simulink model "F16ASYM_Controlled"  (R2015a)
settings: Solver=ode3  SolverMode=SingleTasking  StartTime=0.0  StopTime=inf  FixedStep=T_sim  RelTol=1e-3
InitFcn:
  | load('NN_c_weights_Last_stable.mat')
StopFcn:
  | Final_results
values from neighbouring files (symbols this model uses):
  a1 = fitresult.p1    [Stall_protection.m]
  alpha_map_eval = ones(size(M_eval))*NaN    [Auto_trim_aid.m]    (also in Autotrim_maps.mat = [nan nan 0.277598136245 0.119432432992 0.0579479097061 0.027)
  beta_map_eval = ones(size(M_eval))*NaN    [Auto_trim_aid.m]    (also in Autotrim_maps.mat = [nan nan -0.00151549403324 0.00117807579006 -0.0052086799721)
  C_L_0 = fitresult.p2    [Stall_protection.m]
  G_eval = NaN*ones(size(M_sq,2),size(H_sq,2))    [Stall_protection.m]
  H_sq = unique(sort(H_sq))    [Stall_protection.m]
  H_sq_autotrim = min( F_envelope.H_1g):2000:max(F_envelope.H_1g)    [Auto_trim_aid.m]    (also in Autotrim_maps.mat = [0 2000 4000 6000 8000 10000 12000 14000 16000 18000])
  K_b_q_extrap_ACC = K_b_q_extrap    [RUN_ME.m]
  K_b_q_extrap_AoA = K_b_q_extrap    [RUN_ME.m]
  M_sq = unique(sort(M_sq))    [Stall_protection.m]
  M_sq_autotrim = 0:0.1:max(F_envelope.M_1g)    [Auto_trim_aid.m]    (also in Autotrim_maps.mat = [0 0.1 0.2 0.3 0.4 0.5 0.6 0.7 0.8 0.9 1 1.1 ... (21 element)
  T_sim = 0.02    [RUN_ME.m]
  tau_q_extrap_ACC = tau_q_extrap    [RUN_ME.m]
  tau_q_extrap_AoA = tau_q_extrap    [RUN_ME.m]
  velocity = M_eval(I,J)*a    [Auto_trim_aid.m]
undefined symbols (not defined in the file or in its folder): ACCEL, B, Earth, fi_flag_Simulink, GYRO, H_sq_sche, k_B, K_b_ACC_extrap, K_b_AoA_extrap, latitude, longitude, m, m_B, M_sq_sche, Model_used_flag, rad, s, sigbuilder_block, Stall_curve, tau_ACC_extrap, tau_AoA_extrap, Theta_1_roll_last, Theta_2_roll_last, Theta_3_roll_last, trim_control, trim_state, trim_throttle, V_Comp_A_w_z_last, V_Comp_last, V_Comp_last_ONE, V_long_lastA_w_z, V_long_lastAoA, V_roll_last, V_roll_lastMOD, V_yaw_last, W_Comp_A_w_z_last, W_Comp_last, W_long_lastA_w_z, W_long_lastAoA, W_roll_last, W_roll_lastMOD, W_yaw_last, WGS84
libraries: Adaptive_FaultTolerantControl x57, dspsigops x37, F16_Actuator_Library x14, commnoisgen2 x13, simulink x11, simulink_extras x10, dsparch4 x6, aerolibatmos2 x6, aerolibtransform2 x6, aerolibfltsims x3, dspvision x3, dspsnks4 x3
(part 1 of 14)
Description:
  | This models and controllers were implemented by David Torres Ocaña at Cranfield University
settings Model: ModifiedHistory=This models and controllers were implemented by David Torres Ocaña at Cranfield University  MAModelExclusionFile=C:\Users\David\Documents\Estudios y formación academica\Cranfield\Thesis F16\Work\Solutions\7dof Base\F16ASYM_Controlled_exclusions.xml  Creator=David  LastModifiedBy=david
settings SolverCC: AutoInsertRateTranBlk=on
settings DataIOCC: SaveOutput=off  SignalLogging=off  DSMLogging=off  SaveTime=off
settings OptimizationCC: BlockReduction=off  InlineParams=on  InlineInvariantSignals=on  EnableMemcpy=off  ExpressionDepthLimit=2147483647  StateBitsets=on  DataBitsets=on  ZeroExternalMemoryAtStartup=off  ZeroInternalMemoryAtStartup=off  NoFixptDivByZeroProtection=on  EfficientMapNaN2IntZero=off  OptimizeModelRefInitCode=on  LifeSpan=1
settings DebuggingCC: UnderspecifiedInitializationDetection=Classic  MergeDetectMultiDrivingBlocksExec=none  SolverPrmCheckMsg=warning  ParameterPrecisionLossMsg=none  StateNameClashWarn=warning
settings HardwareCC: ProdIntDivRoundTo=Floor  ProdEndianess=LittleEndian  ProdHWDeviceType=Generic->Custom
settings RTWCC: SystemTargetFile=ert.tlc  TLCOptions=-p0  GenCodeOnly=on  TemplateMakefile=ert_default_tmf  Description=Embedded Coder  GenerateReport=on  RTWVerbose=off  IncludeHyperlinkInReport=on  LaunchReport=on
settings CodeAppCC: ForceParamTrailComments=on  IgnoreCustomStorageClasses=off  SimulinkDataObjDesc=on  CustomSymbolStrGlobalVar=rt$N$M  CustomSymbolStrType=$N$M  CustomSymbolStrFcn=$N$M$F  CustomSymbolStrMacro=$N$M  InsertBlockDesc=on  InternalIdentifier=Classic
settings ERTTargetCC: TargetLangStandard=C99 (ISO)  ParMdlRefBuildCompliant=on  CompOptLevelCompliant=on  ConcurrentExecutionCompliant=on  IncludeMdlTerminateFcn=off  SuppressErrorStatus=on  ERTFirstTimeCompliant=on  SupportAbsoluteTime=off  SupportNonFinite=off  SupportComplex=off  PurelyIntegerCode=on  SupportContinuousTime=off  SupportVariableSizeSignals=off  ModelStepFunctionPrototypeControlCompliant=on  CPPClassGenCompliant=on  RootIOFormat=Structure reference  ERTCustomFileTemplate=example_file_process.tlc

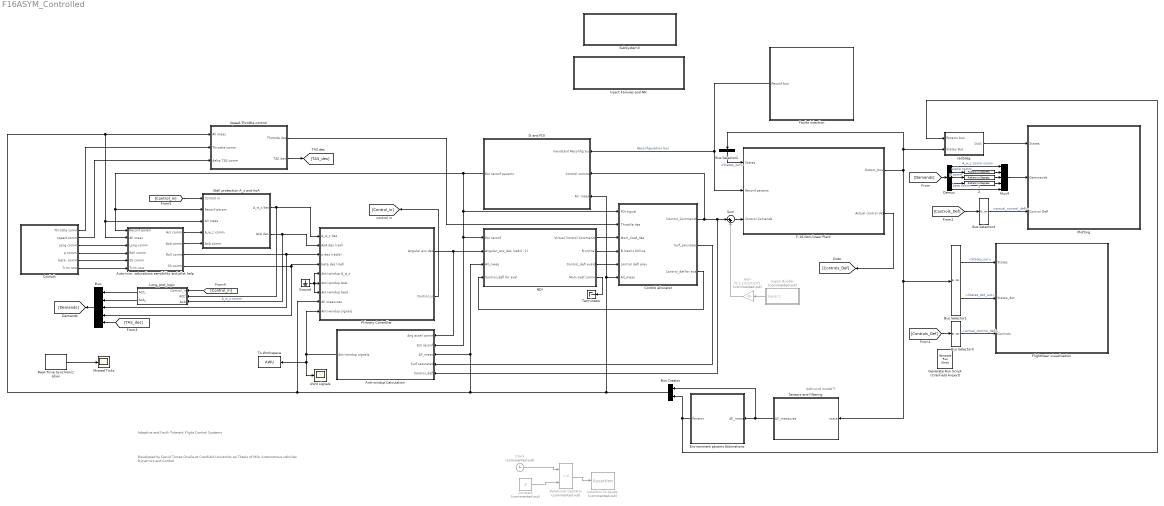
== system F16ASYM_Controlled ==
  note: Developed by David Torres Ocaña
      | at Cranfield University as Thesis of
      | MSc Autonomous vehicles Dynamics and Control
  note: Add wind model??
  note: Adaptive and Fault-Tolerant Flight Control Systems
  "  " : simulink_extras/Transformations/Radians to Degrees
  "  1" : simulink_extras/Transformations/Radians to Degrees
  "  2" : simulink_extras/Transformations/Radians to Degrees
  AWU signals : Scope
      settings: YMin=-30  YMax=15  SaveName=ScopeData20
  Anti-windup Calculation : Subsystem  Variant=on  OverrideUsingVariant=No reconfigurable
  Assertion to pause : Assertion  Commented=on  AssertionFailFcn=|  StopWhenAssertionFail=off
      | set_param(bdroot,'SimulationCommand','pause'),
      | disp(sprintf('\nSimulation paused.'))
  "Auto-trim, saturations sensibility and pilot help" : Subsystem
  Bus Creator : BusCreator  Inputs=2
  Bus Selector1 : BusSelector  OutputSignals=States_out,States_dot_out
  Bus Selector2 : BusSelector  OutputSignals=States_out
  Bus Selector3 : BusSelector  OutputSignals=actual_control_defl
  Bus Selector4 : BusSelector  OutputSignals=actual_control_defl
  Clock : Clock  Commented=on
  Cockpit : Subsystem
      mask Display:
      | image(imread('Cockpit2.jpg'))
      | 
      | port_label('output', 1, 'Throttle comm')
      | port_label('output', 2, 'Speed comm')
      | port_label('output', 3, 'Long comm')
      | port_label('output', 4, 'p comm')
      | port_label('output', 5, 'beta comm')
      | port_label('output', 6, 'Trim now')
  Constant : Constant  Commented=on  Value=5
  Control allocator : Subsystem  Variant=on  OverrideUsingVariant=Control Allocator: NO RECONFIG
  Demux : Demux  Outputs=5
  Environment params Estimations : Subsystem
  F-16 Non-linear Plant : Subsystem  Variant=on  OverrideUsingVariant=Reconfigurable
      mask Display:
      | image(imread('f16.jpg'))
      | 
      | port_label('output', 1, 'Out_bus')
      | port_label('output', 2, 'Actual Control deflec')
      | 
      | port_label('input', 1, 'State_feedback')
      | port_label('input', 2, 'Reconf_params')
      | port_label('input', 3, 'Control_Commands')
      | 
      | % Variant dealing
      | ActiveVar = get_param(gcb,'activevariant');
      | 
      | 
      | disp(['{\bf\fontsize{16}',ActiveVar,'}'], 'texmode','on');
  Faults injection : Subsystem
      settings: OpenFcn=Control_GUI
      mask Display: disp(['{\bf \fontsize{16}',sprintf('Faults \n and\n  deviations\n  injection'),'}'], 'texmode','on');
  FlightGear visualization : Subsystem  TreatAsAtomicUnit=on
      mask Display:
      | % disp('{\bf\fontsize{20} Flight Gear}', 'texmode','on');
      | image(imread('FG F16.jpg'))
      | % image(imread('FlightGear_logo.png'))
  Gain : Gain  Commented=on  Gain=[0,1,1,0,0,0,0,0]
  Generate Run Script (Cranfield Airport) : aerolibfltsims/Generate Run Script  OutputFileName=runfg.bat  FlightGearBaseDirectory=C:\Program Files\FlightGear  GeometryModelName=f16  DestinationPort=5502  OriginAddress=127.0.0.1  OriginPort=5505  LocalAddress=127.0.0.1  AirportId=EGTC  RunwayId=1  InitialAltitude=trim_state(3)*3.2808399  InitialHeading=0  OffsetDistance=4.72  OffsetAzimuth=0  GenerateFile=off  Architecture=Win64  dataFlow=Send
  Ground : Ground
  Inject Failures and NN : Subsystem
      settings: OpenFcn=Control_GUI
      mask Display: disp('Inject Failures & NN management GUI')
  Long_plot_logic : MATLAB Function  TreatAsAtomicUnit=on
  Missed Ticks : Scope
      settings: TickLabels=on  TimeRange=20  YMin=0  YMax=70  SaveName=ScopeData29
  Mux : Mux  Inputs=[1 1 1 1 1]
  Mux4 : Mux  Inputs=5
  NDI : Subsystem  Variant=on  OverrideUsingVariant=NDI: NO RECONFIG
  Plotting : Subsystem
      mask Display:
      | disp('{\bf\fontsize{20} Plotting}', 'texmode','on');
      | % port_label('input', 1, 'States')
      | % port_label('input', 2, 'Demans')
  Primary Controller : Subsystem  Variant=on  OverrideUsingVariant=Adaptive Controller Crossed+AWU+Lim
  Real-Time Synchronization : sldrtlib/Real-Time Synchronization  SampleTime=T_sim  MaxMissedTicks=100000  ShowMissedTicks=on  YieldWhenWaiting=on
  Relational Operator : RelationalOperator  Commented=on  Operator=~=  OutDataTypeStr=boolean
  SI and FDI : Subsystem  Variant=on  OverrideUsingVariant=Realistic
      mask Display:
      | % Variant dealing
      | ActiveVar = get_param(gcb,'activevariant');
      | 
      | 
      | 
      | disp(['{\bf \fontsize{14}',sprintf('SI \n&\nFDI\n\n '),ActiveVar,'}'], 'texmode','on');
  Sensors and filtering : Subsystem  Variant=on  OverrideUsingVariant=No noise
  Signal Builder : Subsystem  Tag=STV Subsys  Commented=on  LoadFcn=sigbuilder_block('load');  StartFcn=sigbuilder_block('start');  StopFcn=sigbuilder_block('stop');  ClipboardFcn=sigbuilder_block('clipboard');  mask(Sigbuilder block){}
      mask help: Simulink:masks:SigbuilderBlock_MD
      mask init:
      | if ~strcmp(get_param(bdroot(gcbh),'SimulationStatus'),'stopped') tuvar = sigbuilder_block('maskInit'); end
      settings: CopyFcn=sigbuilder_block('copy');  DeleteFcn=sigbuilder_block('delete');  ModelCloseFcn=sigbuilder_block('modelClose');  PreSaveFcn=sigbuilder_block('preSave');  PauseFcn=sigbuilder_block('pause');  ContinueFcn=sigbuilder_block('continue');  NameChangeFcn=sigbuilder_block('namechange');  OpenFcn=sigbuilder_block('open',[437.25 118.5 550.5 394.5 ]);  CloseFcn=sigbuilder_block('close');
      mask Display: plot(0, 0, 100, 100,[2, 2, 32, 32, 2], [68, 8, 8, 68, 68],[32, 2], [38, 38], [32, 19, 2],[53, 60, 44], [32, 17, 17, 2],[16, 16, 31, 31]);txt = getActiveGroup(gcbh);text(2, 100, txt,'verticalAlignment', 'top');
  Speed-Throttle control : Subsystem
  Stall protection A_z and AoA : Subsystem  Variant=on  OverrideUsingVariant=Using AoA
  SubSystem3 : Subsystem
      settings: OpenFcn=FE_plot
      mask Display:
      | % image(imread('FE.png'))
      | 
      | disp('Flight Envelope position');
  Sum : Sum  Inputs=|++
  Terminator : Terminator
  To Workspace : ToWorkspace  VariableName=AWU  SaveFormat=Timeseries  SampleTime=-1
  rad2deg : Subsystem
  wires:
  rad2deg/1(Out1) -> Plotting/1(States)
  F-16 Non-linear Plant/1(Output_bus) -> Bus Selector1/1, Sensors and filtering/1(state), Bus Selector2/1, rad2deg/2(States Bus)
  Bus Selector1/1 -> FlightGear visualization/1(States)  "<States_out>"
  Bus Selector1/2 -> FlightGear visualization/2(States_dot)  "<States_dot_out>"
  [Demands] -> Demux/1
  Sensors and filtering/1(All_measures) -> Bus Creator/1, Environment params Estimations/1(All_meas)
  Environment params Estimations/1(Params) -> Bus Creator/2, rad2deg/1(Params bus)
  Demux/3 -> "  1"/1  "p comm"
  Demux/4 -> "  2"/1  "beta comm"
  Demux/2 -> "  "/1  "alpha comm"
  [Controls_Def] -> Bus Selector3/1
  Control allocator/2(Surf_saturated) -> Anti-windup Calculation/4(Surf saturated)
  NDI/1(Virtual Control Commands) -> Control allocator/3(Mom_Coef_des)
  Ground/1 -> Primary Controller/7(Anti-windup beta), Primary Controller/5(Anti-windup A_w_z), Primary Controller/6(Anti-windup AoA)
  Mux4/1 -> Plotting/2(Demmands)
  Bus Selector2/1 -> F-16 Non-linear Plant/1(States)  "<States_out>"
  NDI/2(B online) -> Control allocator/4(B matrix Online)
  Demux/1 -> Mux4/1  "A_w_z comm comm"
  "  "/1 -> Mux4/2
  "  1"/1 -> Mux4/3
  "  2"/1 -> Mux4/4
  F-16 Non-linear Plant/2(Actual control def) -> [Controls_Def]
  Bus Selector3/1 -> FlightGear visualization/3(Controls)  "<actual_control_defl>"
  Primary Controller/1(Angular acc des) -> NDI/2(Angular_acc_des (rad/s^2)), Anti-windup Calculation/1(Ang accel comm)
  NDI/3(Control_defl evald) -> Control allocator/5(control defl prev)
  Control allocator/3(Control_def for eval) -> NDI/4(Control_defl for eval)
  [Controls_Def] -> Bus Selector4/1
  Bus Selector4/1 -> Plotting/3(Control Defl)  "<actual_control_defl>"
  Demux/5 -> Mux4/5
  Faults injection/1(Reconf bus) -> F-16 Non-linear Plant/2(Reconf params), SI and FDI/1(Inexistent Reconfig bus)  "Reconfiguration bus"
  Bus Creator/1 -> SI and FDI/3(All  meas), Control allocator/6(All_meas), NDI/3(All_meas), Anti-windup Calculation/3(All_meas), Primary Controller/8(All measures), "Auto-trim, saturations sensibility and pilot help"/2(All meas), Stall protection A_z and AoA/3(All meas), Speed-Throttle control/1(All meas)
  "Auto-trim, saturations sensibility and pilot help"/1(Acc comm) -> Stall protection A_z and AoA/4(A_w_z comm)
  Anti-windup Calculation/1(Anti-windup signals) -> To Workspace/1, AWU signals/1, Primary Controller/9(Anti-windup signals)
  Stall protection A_z and AoA/1(A_w_z des) -> Primary Controller/1(A_w_z des), Long_plot_logic/2(ACC)  "A_w_z comm"
  Stall protection A_z and AoA/2(AoA des) -> Long_plot_logic/3(AoA), Primary Controller/2(AoA des (rad))
  "Auto-trim, saturations sensibility and pilot help"/4("SS comm ") -> Primary Controller/4(beta des (rad)), Mux/4
  "Auto-trim, saturations sensibility and pilot help"/3("Roll comm ") -> Mux/3, Primary Controller/3(p des (rad/s))
  SI and FDI/1(Est reconf params) -> "Auto-trim, saturations sensibility and pilot help"/1(Reconf param), Stall protection A_z and AoA/2(Reconf param), Anti-windup Calculation/2(Est reconf), NDI/1(Est reconf), Control allocator/1(FDI signal)
  Real-Time Synchronization/1 -> Missed Ticks/1
  Cockpit/3(Long comm) -> "Auto-trim, saturations sensibility and pilot help"/3(Long comm)
  Cockpit/4(p comm) -> "Auto-trim, saturations sensibility and pilot help"/4(Roll comm)
  Cockpit/5(beta  comm) -> "Auto-trim, saturations sensibility and pilot help"/5(SS comm)
  "Auto-trim, saturations sensibility and pilot help"/2(AoA comm) -> Stall protection A_z and AoA/5(AoA comm)
  Cockpit/1(Throttle comm) -> Speed-Throttle control/2(Throttle comm)
  Cockpit/2(speed comm) -> Speed-Throttle control/3(delta TAS comm)
  Speed-Throttle control/1(Throttle des) -> Control allocator/2(Throttle des)
  Mux/1 -> [Demands]
  Speed-Throttle control/2(TAS des) -> [TAS_des]
  [TAS_des] -> Mux/5
  Primary Controller/2(Control_in) -> [Control_in]
  [Control_in] -> Long_plot_logic/1(Control_in)
  Long_plot_logic/1(ACC_) -> Mux/1
  Long_plot_logic/2(AoA_) -> Mux/2
  [Control_in] -> Stall protection A_z and AoA/1(Control in)
  NDI/4(Mom coef comm) -> Terminator/1
  Signal Builder/1(Signal 1) -> Gain/1
  Control allocator/1(Control_Commands) -> SI and FDI/2(Control comms), Anti-windup Calculation/5(Control_defl), Sum/1
  Cockpit/6(Trim now) -> "Auto-trim, saturations sensibility and pilot help"/6(Trim now)
  Sum/1 -> F-16 Non-linear Plant/3(Control Comands)
  Gain/1 -> Sum/2
  Relational Operator/1 -> Assertion to pause/1
  Clock/1 -> Relational Operator/1
  Constant/1 -> Relational Operator/2

== system F16ASYM_Controlled/Anti-windup Calculation ==
  Ang accel comm : Inport
  Est reconf : Inport  Port=2
  All_meas : Inport  Port=3
  Surf saturated : Inport  Port=4
  Control_defl : Inport  Port=5
  Anti-windup: NO reconfigurable : Subsystem  VariantControl=No reconfigurable
  Anti-windup: Reconfigurable : Subsystem  VariantControl=Reconfigurable
  Anti-windup signals : Outport

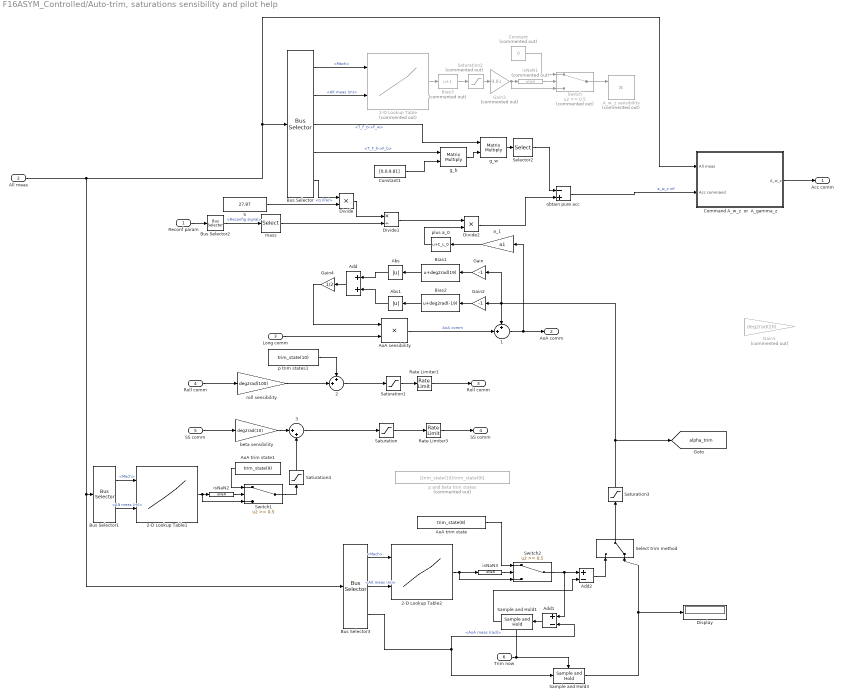
== system F16ASYM_Controlled/Auto-trim, saturations sensibility and pilot help ==
  Reconf param : Inport
  All meas : Inport  Port=2
  Long comm : Inport  Port=3
  Roll comm : Inport  Port=4
  SS comm : Inport  Port=5
  Trim now : Inport  Port=6
  " 1" : Sum  Inputs=++|
  " 2" : Sum  Inputs=++|
  " 3" : Sum  Inputs=|++
  2-D Lookup Table : Lookup_n-D  Commented=on  BreakpointsForDimension1=M_sq  BreakpointsForDimension2=H_sq  Table=G_eval  RemoveProtectionInput=on  SampleTime=5*T_sim  RndMeth=Simplest  InputSameDT=on
  2-D Lookup Table1 : Lookup_n-D  BreakpointsForDimension1=M_sq_autotrim  BreakpointsForDimension2=H_sq_autotrim  Table=beta_map_eval  ExtrapMethod=Clip  RemoveProtectionInput=on  UseLastTableValue=on  SampleTime=2*T_sim  RndMeth=Simplest  InputSameDT=on
  2-D Lookup Table2 : Lookup_n-D  BreakpointsForDimension1=M_sq_autotrim  BreakpointsForDimension2=H_sq_autotrim  Table=alpha_map_eval  ExtrapMethod=Clip  RemoveProtectionInput=on  UseLastTableValue=on  SampleTime=2*T_sim  RndMeth=Simplest  InputSameDT=on
  A_w_z sensibility : Product  Commented=on  Inputs=**
  Abs : Abs
  Abs1 : Abs
  Add : Sum
  Add1 : Sum  Inputs=+-
  Add2 : Sum  Inputs=+-
  AoA sensibility : Product  Inputs=**
  AoA trim state : Constant  Value=trim_state(8)
  AoA trim state1 : Constant  Value=trim_state(9)
  Bias1 : Bias  Bias=deg2rad(19)
  Bias2 : Bias  Bias=deg2rad(-19)
  Bias3 : Bias  Commented=on  Bias=1
  Bus Selector : BusSelector  OutputSignals=signal2.Mach,signal1.Alt meas (m),signal2.T_F_b->F_w,signal2.T_F_h->F_b,signal2.q (Pa)
  Bus Selector1 : BusSelector  OutputSignals=signal2.Mach,signal1.Alt meas (m)
  Bus Selector2 : BusSelector  OutputSignals=Reconfig signal
  Bus Selector3 : BusSelector  OutputSignals=signal2.Mach,signal1.Alt meas (m),signal1.AoA meas (rad)
  Command A_w_z  or  A_gamma_z : Subsystem  mask{Crit=A_w_z, Criteria=0}
      mask prompts: Crit "Commdn in:"
      mask init:
      | val = get_param(gcb,'MaskValues');
      | switch lower(val{1})
      |  case 'A_w_z'
      |      Criteria=0;
      |  case 'A_gamma_z'
      |      Criteria=1;
      | end
      mask TypeOptions Crit: A_w_z | A_gamma_z
      mask Display:
      | val = get_param(gcb,'MaskValues');
      | 
      | disp(['{\bf\fontsize{16}',upper(val{1}),'}'], 'texmode','on');
  Constant : Constant  Commented=on  Value=0
  Constant1 : Constant  Value=[0,0,9.81]
  Display : Display
  Divide : Product  Inputs=**
  Divide1 : Product  Inputs=*/
  Divide2 : Product  Inputs=**
  Gain : Gain  Gain=-1
  Gain1 : Gain  Commented=on  Gain=deg2rad(20)
  Gain2 : Gain  Gain=-1
  Gain3 : Gain  Commented=on  Gain=9.81
  Gain4 : Gain  Gain=1/2
  Rate Limiter1 : RateLimiter  RisingSlewLimit=deg2rad(200)  FallingSlewLimit=-deg2rad(200)  SampleTimeMode=inherited  InitialCondition=trim_state(10)
  Rate Limiter3 : RateLimiter  RisingSlewLimit=deg2rad(15)  FallingSlewLimit=-deg2rad(15)  SampleTimeMode=inherited  InitialCondition=trim_state(9)
  S : Constant  Value=27.87
  Sample and Hold1 : dspsigops/Sample and Hold  trig=Either edge  initCond=0  latchinput=off
  Sample and Hold3 : dspsigops/Sample and Hold  trig=Either edge  initCond=trim_state(8)  latchinput=off
  Saturation : Saturate  UpperLimit=deg2rad(10)  LowerLimit=deg2rad(-10)
  Saturation1 : Saturate  UpperLimit=deg2rad(100)  LowerLimit=deg2rad(-100)
  Saturation2 : Saturate  Commented=on  UpperLimit=9  LowerLimit=0
  Saturation3 : Saturate  UpperLimit=deg2rad(17)  LowerLimit=deg2rad(0)
  Saturation4 : Saturate  UpperLimit=deg2rad(10)  LowerLimit=deg2rad(-10)
  Select trim method : ManualSwitch  CurrentSetting=0
  Selector2 : Selector  InputPortWidth=3  Indices=3
  Switch : Switch  Commented=on  Threshold=0.5
  Switch1 : Switch  Threshold=0.5
  Switch2 : Switch  Threshold=0.5
  a_1 : Gain  Gain=a1
  beta sensibility : Gain  Gain=deg2rad(10)
  g_b : Product  Multiplication=Matrix(*)
  g_w : Product  Multiplication=Matrix(*)
  isNaN1 : RelationalOperator  Commented=on  Operator=isNaN  OutDataTypeStr=boolean
  isNaN2 : RelationalOperator  Operator=isNaN  OutDataTypeStr=boolean
  isNaN3 : RelationalOperator  Operator=isNaN  OutDataTypeStr=boolean
  mass : Selector  InputPortWidth=19
  obtain pure acc : Sum  Inputs=-+
  p and beta trim states : Constant  Commented=on  Value=[trim_state(10);trim_state(9)]
  p trim states1 : Constant  Value=trim_state(10)
  plus a_0 : Bias  Bias=C_L_0
  roll sensibility : Gain  Gain=deg2rad(100)
  Acc comm : Outport
  AoA comm : Outport  Port=2
  "Roll comm " : Outport  Port=3
  "SS comm " : Outport  Port=4
  tag scope: alpha_trim=global
  wires:
  SS comm/1 -> beta sensibility/1
  Roll comm/1 -> roll sensibility/1
  Rate Limiter3/1 -> "SS comm "/1
  Rate Limiter1/1 -> "Roll comm "/1
  Saturation/1 -> Rate Limiter3/1
  Saturation1/1 -> Rate Limiter1/1
  Command A_w_z  or  A_gamma_z/1(A_w_z) -> Acc comm/1
  Reconf param/1 -> Bus Selector2/1
  " 1"/1 -> a_1/1, AoA comm/1
  Select trim method/1 -> Saturation3/1
  Bus Selector/1 -> 2-D Lookup Table/1  "<Mach>"
  Bus Selector/2 -> 2-D Lookup Table/2  "<Alt meas (m)>"
  2-D Lookup Table/1 -> Bias3/1
  Switch/1 -> A_w_z sensibility/1
  Long comm/1 -> AoA sensibility/2
  " 3"/1 -> Saturation/1
  " 2"/1 -> Saturation1/1
  AoA sensibility/1 -> " 1"/2  "AoA comm"
  Gain/1 -> Bias1/1
  Gain2/1 -> Bias2/1
  Bias1/1 -> Abs/1
  Bias2/1 -> Abs1/1
  Abs/1 -> Add/1
  Abs1/1 -> Add/2
  Constant/1 -> Switch/1
  isNaN1/1 -> Switch/2
  Gain3/1 -> isNaN1/1, Switch/3
  Saturation2/1 -> Gain3/1
  Bias3/1 -> Saturation2/1
  p trim states1/1 -> " 2"/1
  All meas/1 -> Command A_w_z  or  A_gamma_z/1(All meas), Bus Selector/1, Bus Selector1/1, Bus Selector3/1
  Bus Selector1/1 -> 2-D Lookup Table1/1  "<Mach>"
  Bus Selector1/2 -> 2-D Lookup Table1/2  "<Alt meas (m)>"
  Bus Selector3/2 -> 2-D Lookup Table2/2  "<Alt meas (m)>"
  Bus Selector3/1 -> 2-D Lookup Table2/1  "<Mach>"
  isNaN2/1 -> Switch1/2
  2-D Lookup Table1/1 -> Switch1/3, isNaN2/1
  AoA trim state/1 -> Switch2/1
  isNaN3/1 -> Switch2/2
  2-D Lookup Table2/1 -> Switch2/3, isNaN3/1
  Switch1/1 -> Saturation4/1
  beta sensibility/1 -> " 3"/1
  roll sensibility/1 -> " 2"/2
  Saturation3/1 -> " 1"/1, Gain/1, Gain2/1, [alpha_trim]
  Bus Selector2/1 -> mass/1  "<Reconfig signal>"
  Divide/1 -> Divide1/1
  mass/1 -> Divide1/2
  S/1 -> Divide/2
  Bus Selector/5 -> Divide/1  "<q (Pa)>"
  a_1/1 -> plus a_0/1
  Divide1/1 -> Divide2/1
  plus a_0/1 -> Divide2/2
  Bus Selector/3 -> g_w/1  "<T_F_b->F_w>"
  Bus Selector/4 -> g_b/1  "<T_F_h->F_b>"
  Constant1/1 -> g_b/2
  g_b/1 -> g_w/2
  g_w/1 -> Selector2/1
  obtain pure acc/1 -> Command A_w_z  or  A_gamma_z/2(Acc command)  "a_w_z inf"
  Divide2/1 -> obtain pure acc/2
  Selector2/1 -> obtain pure acc/1
  Add/1 -> Gain4/1
  Gain4/1 -> AoA sensibility/1
  Bus Selector3/3 -> Add1/2, Sample and Hold3/1  "<AoA meas (rad)>"
  Sample and Hold3/1 -> Display/1, Select trim method/2
  Switch2/1 -> Add2/1, Add1/1
  Add2/1 -> Select trim method/1
  Trim now/1 -> Sample and Hold3/Trigger, Sample and Hold1/Trigger
  Add1/1 -> Sample and Hold1/1
  Sample and Hold1/1 -> Add2/2
  AoA trim state1/1 -> Switch1/1
  Saturation4/1 -> " 3"/2

== system F16ASYM_Controlled/Cockpit ==
  note: Command generation
  Delay : Delay  Commented=on  DelayLength=floor(10/T_sim)
  Delay1 : Delay  Commented=on  DelayLength=floor(5/T_sim)
  Delay2 : Delay  Commented=on  DelayLength=floor(10/T_sim)
  Delay3 : Delay  Commented=on  DelayLength=floor(5/T_sim)
  Delay4 : Delay  Commented=on  DelayLength=floor(10/T_sim)
  Delay5 : Delay  Commented=on  DelayLength=floor(5/T_sim)
  Delay6 : Delay  DelayLength=floor(30/T_sim)
  Delay7 : Delay  DelayLength=floor(25/T_sim)
  Delay8 : Delay  DelayLength=floor(10/T_sim)
  Demux2 : Demux  Outputs=3
  Joystick : Subsystem  Commented=on
  Manual Switch1 : ManualSwitch  CurrentSetting=0
  Mux{1,3..7} (6 alike) : Mux  Commented=on  Inputs=3
  Mux2 : Mux  Inputs=3
  Mux8 : Mux  Inputs=3
  Mux9 : Mux  Inputs=3
  Signal Builder : Subsystem  Tag=STV Subsys  Commented=on  LoadFcn=sigbuilder_block('load');  StartFcn=sigbuilder_block('start');  StopFcn=sigbuilder_block('stop');  ClipboardFcn=sigbuilder_block('clipboard');  mask(Sigbuilder block){}
      mask help: Simulink:masks:SigbuilderBlock_MD
      mask init:
      | if ~strcmp(get_param(bdroot(gcbh),'SimulationStatus'),'stopped') tuvar = sigbuilder_block('maskInit'); end
      settings: CopyFcn=sigbuilder_block('copy');  DeleteFcn=sigbuilder_block('delete');  ModelCloseFcn=sigbuilder_block('modelClose');  PreSaveFcn=sigbuilder_block('preSave');  PauseFcn=sigbuilder_block('pause');  ContinueFcn=sigbuilder_block('continue');  NameChangeFcn=sigbuilder_block('namechange');  OpenFcn=sigbuilder_block('open',[6 28.5 1012.5 484.5 ]);  CloseFcn=sigbuilder_block('close');
      mask Display: plot(0, 0, 100, 100,[2, 2, 32, 32, 2], [68, 8, 8, 68, 68],[32, 2], [38, 38], [32, 19, 2],[53, 60, 44], [32, 17, 17, 2],[16, 16, 31, 31]);txt = getActiveGroup(gcbh);text(2, 100, txt,'verticalAlignment', 'top');
  Signal Builder1 : Subsystem  Tag=STV Subsys  Commented=on  LoadFcn=sigbuilder_block('load');  StartFcn=sigbuilder_block('start');  StopFcn=sigbuilder_block('stop');  ClipboardFcn=sigbuilder_block('clipboard');  mask(Sigbuilder block){}
      mask help: Simulink:masks:SigbuilderBlock_MD
      mask init:
      | if ~strcmp(get_param(bdroot(gcbh),'SimulationStatus'),'stopped') tuvar = sigbuilder_block('maskInit'); end
      settings: CopyFcn=sigbuilder_block('copy');  DeleteFcn=sigbuilder_block('delete');  ModelCloseFcn=sigbuilder_block('modelClose');  PreSaveFcn=sigbuilder_block('preSave');  PauseFcn=sigbuilder_block('pause');  ContinueFcn=sigbuilder_block('continue');  NameChangeFcn=sigbuilder_block('namechange');  OpenFcn=sigbuilder_block('open',[6 28.5 1012.5 484.5 ]);  CloseFcn=sigbuilder_block('close');
      mask Display: plot(0, 0, 100, 100,[2, 2, 32, 32, 2], [68, 8, 8, 68, 68],[32, 2], [38, 38], [32, 19, 2],[53, 60, 44], [32, 17, 17, 2],[16, 16, 31, 31]);txt = getActiveGroup(gcbh);text(2, 100, txt,'verticalAlignment', 'top');
  Signal Builder2 : Subsystem  Tag=STV Subsys  Commented=on  LoadFcn=sigbuilder_block('load');  StartFcn=sigbuilder_block('start');  StopFcn=sigbuilder_block('stop');  ClipboardFcn=sigbuilder_block('clipboard');  mask(Sigbuilder block){}
      mask help: Simulink:masks:SigbuilderBlock_MD
      mask init:
      | if ~strcmp(get_param(bdroot(gcbh),'SimulationStatus'),'stopped') tuvar = sigbuilder_block('maskInit'); end
      settings: CopyFcn=sigbuilder_block('copy');  DeleteFcn=sigbuilder_block('delete');  ModelCloseFcn=sigbuilder_block('modelClose');  PreSaveFcn=sigbuilder_block('preSave');  PauseFcn=sigbuilder_block('pause');  ContinueFcn=sigbuilder_block('continue');  NameChangeFcn=sigbuilder_block('namechange');  OpenFcn=sigbuilder_block('open',[6 28.5 1012.5 484.5 ]);  CloseFcn=sigbuilder_block('close');
      mask Display: plot(0, 0, 100, 100,[2, 2, 32, 32, 2], [68, 8, 8, 68, 68],[32, 2], [38, 38], [32, 19, 2],[53, 60, 44], [32, 17, 17, 2],[16, 16, 31, 31]);txt = getActiveGroup(gcbh);text(2, 100, txt,'verticalAlignment', 'top');
  Signal Builder3 : Subsystem  Tag=STV Subsys  Commented=on  LoadFcn=sigbuilder_block('load');  StartFcn=sigbuilder_block('start');  StopFcn=sigbuilder_block('stop');  ClipboardFcn=sigbuilder_block('clipboard');  mask(Sigbuilder block){}
      mask help: Simulink:masks:SigbuilderBlock_MD
      mask init:
      | if ~strcmp(get_param(bdroot(gcbh),'SimulationStatus'),'stopped') tuvar = sigbuilder_block('maskInit'); end
      settings: CopyFcn=sigbuilder_block('copy');  DeleteFcn=sigbuilder_block('delete');  ModelCloseFcn=sigbuilder_block('modelClose');  PreSaveFcn=sigbuilder_block('preSave');  PauseFcn=sigbuilder_block('pause');  ContinueFcn=sigbuilder_block('continue');  NameChangeFcn=sigbuilder_block('namechange');  OpenFcn=sigbuilder_block('open',[6 28.5 1012.5 484.5 ]);  CloseFcn=sigbuilder_block('close');
      mask Display: plot(0, 0, 100, 100,[2, 2, 32, 32, 2], [68, 8, 8, 68, 68],[32, 2], [38, 38], [32, 19, 2],[53, 60, 44], [32, 17, 17, 2],[16, 16, 31, 31]);txt = getActiveGroup(gcbh);text(2, 100, txt,'verticalAlignment', 'top');
  Signal Builder4 : Subsystem  Tag=STV Subsys  Commented=on  LoadFcn=sigbuilder_block('load');  StartFcn=sigbuilder_block('start');  StopFcn=sigbuilder_block('stop');  ClipboardFcn=sigbuilder_block('clipboard');  mask(Sigbuilder block){}
      mask help: Simulink:masks:SigbuilderBlock_MD
      mask init:
      | if ~strcmp(get_param(bdroot(gcbh),'SimulationStatus'),'stopped') tuvar = sigbuilder_block('maskInit'); end
      settings: CopyFcn=sigbuilder_block('copy');  DeleteFcn=sigbuilder_block('delete');  ModelCloseFcn=sigbuilder_block('modelClose');  PreSaveFcn=sigbuilder_block('preSave');  PauseFcn=sigbuilder_block('pause');  ContinueFcn=sigbuilder_block('continue');  NameChangeFcn=sigbuilder_block('namechange');  OpenFcn=sigbuilder_block('open',[6 28.5 1012.5 484.5 ]);  CloseFcn=sigbuilder_block('close');
      mask Display: plot(0, 0, 100, 100,[2, 2, 32, 32, 2], [68, 8, 8, 68, 68],[32, 2], [38, 38], [32, 19, 2],[53, 60, 44], [32, 17, 17, 2],[16, 16, 31, 31]);txt = getActiveGroup(gcbh);text(2, 100, txt,'verticalAlignment', 'top');
  Signal Builder5 : Subsystem  Tag=STV Subsys  Commented=on  LoadFcn=sigbuilder_block('load');  StartFcn=sigbuilder_block('start');  StopFcn=sigbuilder_block('stop');  ClipboardFcn=sigbuilder_block('clipboard');  mask(Sigbuilder block){}
      mask help: Simulink:masks:SigbuilderBlock_MD
      mask init:
      | if ~strcmp(get_param(bdroot(gcbh),'SimulationStatus'),'stopped') tuvar = sigbuilder_block('maskInit'); end
      settings: CopyFcn=sigbuilder_block('copy');  DeleteFcn=sigbuilder_block('delete');  ModelCloseFcn=sigbuilder_block('modelClose');  PreSaveFcn=sigbuilder_block('preSave');  PauseFcn=sigbuilder_block('pause');  ContinueFcn=sigbuilder_block('continue');  NameChangeFcn=sigbuilder_block('namechange');  OpenFcn=sigbuilder_block('open',[6 28.5 1012.5 484.5 ]);  CloseFcn=sigbuilder_block('close');
      mask Display: plot(0, 0, 100, 100,[2, 2, 32, 32, 2], [68, 8, 8, 68, 68],[32, 2], [38, 38], [32, 19, 2],[53, 60, 44], [32, 17, 17, 2],[16, 16, 31, 31]);txt = getActiveGroup(gcbh);text(2, 100, txt,'verticalAlignment', 'top');
  Signal Builder6 : Subsystem  Tag=STV Subsys  LoadFcn=sigbuilder_block('load');  StartFcn=sigbuilder_block('start');  StopFcn=sigbuilder_block('stop');  ClipboardFcn=sigbuilder_block('clipboard');  mask(Sigbuilder block){}
      mask help: Simulink:masks:SigbuilderBlock_MD
      mask init:
      | if ~strcmp(get_param(bdroot(gcbh),'SimulationStatus'),'stopped') tuvar = sigbuilder_block('maskInit'); end
      settings: CopyFcn=sigbuilder_block('copy');  DeleteFcn=sigbuilder_block('delete');  ModelCloseFcn=sigbuilder_block('modelClose');  PreSaveFcn=sigbuilder_block('preSave');  PauseFcn=sigbuilder_block('pause');  ContinueFcn=sigbuilder_block('continue');  NameChangeFcn=sigbuilder_block('namechange');  OpenFcn=sigbuilder_block('open',[6 28.5 1012.5 484.5 ]);  CloseFcn=sigbuilder_block('close');
      mask Display: plot(0, 0, 100, 100,[2, 2, 32, 32, 2], [68, 8, 8, 68, 68],[32, 2], [38, 38], [32, 19, 2],[53, 60, 44], [32, 17, 17, 2],[16, 16, 31, 31]);txt = getActiveGroup(gcbh);text(2, 100, txt,'verticalAlignment', 'top');
  Signal Builder7 : Subsystem  Tag=STV Subsys  LoadFcn=sigbuilder_block('load');  StartFcn=sigbuilder_block('start');  StopFcn=sigbuilder_block('stop');  ClipboardFcn=sigbuilder_block('clipboard');  mask(Sigbuilder block){}
      mask help: Simulink:masks:SigbuilderBlock_MD
      mask init:
      | if ~strcmp(get_param(bdroot(gcbh),'SimulationStatus'),'stopped') tuvar = sigbuilder_block('maskInit'); end
      settings: CopyFcn=sigbuilder_block('copy');  DeleteFcn=sigbuilder_block('delete');  ModelCloseFcn=sigbuilder_block('modelClose');  PreSaveFcn=sigbuilder_block('preSave');  PauseFcn=sigbuilder_block('pause');  ContinueFcn=sigbuilder_block('continue');  NameChangeFcn=sigbuilder_block('namechange');  OpenFcn=sigbuilder_block('open',[6 28.5 1012.5 484.5 ]);  CloseFcn=sigbuilder_block('close');
      mask Display: plot(0, 0, 100, 100,[2, 2, 32, 32, 2], [68, 8, 8, 68, 68],[32, 2], [38, 38], [32, 19, 2],[53, 60, 44], [32, 17, 17, 2],[16, 16, 31, 31]);txt = getActiveGroup(gcbh);text(2, 100, txt,'verticalAlignment', 'top');
  Signal Generator : SignalGenerator  Commented=on  WaveForm=square  Amplitude=5  Frequency=0.05
  Sum{,1..5} (6 alike) : Sum  Commented=on  Inputs=|++
  Sum6 : Sum  Inputs=|++
  Sum7 : Sum  Inputs=|++
  deg2rad1 : Gain  Commented=on  Gain=pi/180
  sensibility smooth{1..4} (4 alike) : Fcn  Expr=u(1)^3
  Throttle comm : Outport
  speed comm : Outport  Port=2
  Long comm : Outport  Port=3
  p comm : Outport  Port=4
  beta  comm : Outport  Port=5
  Trim now : Outport  Port=6
  wires:
  Manual Switch1/1 -> Demux2/1
  Joystick/5(sideslip) -> Mux2/3
  Joystick/4(Roll) -> Mux2/2
  Joystick/2(Throttle) -> Throttle comm/1
  Joystick/3(Long: Acc) -> Mux2/1
  Signal Builder/2(Signal 2) -> Mux1/2
  Signal Builder/3(Signal 3) -> Mux1/3
  Joystick/1(speed des) -> speed comm/1
  Demux2/2 -> sensibility smooth1/1  "p comm"
  Demux2/3 -> sensibility smooth2/1  "beta comm"
  Demux2/1 -> sensibility smooth3/1
  sensibility smooth2/1 -> beta  comm/1
  Joystick/6(Trim now) -> Trim now/1
  Signal Generator/1 -> deg2rad1/1
  Sum1/1 -> Delay/1, Sum/1
  Signal Builder1/2(Signal 2) -> Mux3/2
  Signal Builder1/3(Signal 3) -> Mux3/3
  Mux3/1 -> Delay1/1
  Mux1/1 -> Sum1/1
  Delay1/1 -> Sum1/2
  Delay/1 -> Sum/2
  Signal Builder2/2(Signal 2) -> Mux4/2
  Signal Builder2/3(Signal 3) -> Mux4/3
  Signal Builder2/1(Signal 1) -> Mux4/1
  Sum3/1 -> Sum2/1, Delay2/1
  Signal Builder3/2(Signal 2) -> Mux5/2
  Signal Builder3/3(Signal 3) -> Mux5/3
  Mux5/1 -> Delay3/1
  Mux4/1 -> Sum3/1
  Signal Builder3/1(Signal 1) -> Mux5/1
  Delay3/1 -> Sum3/2
  sensibility smooth3/1 -> Long comm/1
  Signal Builder4/2(Signal 2) -> Mux6/2
  Signal Builder4/3(Signal 3) -> Mux6/3
  Signal Builder4/1(Signal 1) -> Mux6/1
  Sum5/1 -> Sum4/1, Delay4/1
  Signal Builder5/2(Signal 2) -> Mux7/2
  Signal Builder5/3(Signal 3) -> Mux7/3
  Mux7/1 -> Delay5/1
  Mux6/1 -> Sum5/1
  Signal Builder5/1(Signal 1) -> Mux7/1
  Delay5/1 -> Sum5/2
  ? -> Mux8/2
  Signal Builder6/3(Signal 3) -> Mux8/3
  Signal Builder6/2(Signal 2) -> Mux8/1
  Sum7/1 -> Sum6/1, Delay7/1
  ? -> Mux9/2
  Signal Builder7/3(Signal 3) -> Mux9/3
  Mux9/1 -> Delay8/1
  Mux8/1 -> Sum7/1
  Signal Builder7/2(Signal 2) -> Mux9/1
  Delay8/1 -> Sum7/2
  Delay7/1 -> Sum6/2
  Sum6/1 -> Delay6/1
  sensibility smooth1/1 -> p comm/1
  Mux2/1 -> Manual Switch1/1
  Delay6/1 -> Manual Switch1/2

== system F16ASYM_Controlled/Control allocator ==
  FDI signal : Inport
  Throttle des : Inport  Port=2
  Mom_Coef_des : Inport  Port=3
  B matrix Online : Inport  Port=4
  control defl prev : Inport  Port=5
  All_meas : Inport  Port=6
  Control allocator: NO RECONF : Subsystem  RTWFcnName=abc  RTWFileName=asas  VariantControl=Control Allocator: NO RECONFIG
      settings: MinAlgLoopOccurrences=on  RTWFcnNameOpts=User specified  RTWFileNameOpts=User specified
  Control allocator: RECONFIG : Subsystem  RTWFcnName=abc  RTWFileName=asas  VariantControl=Control Allocator: RECONFIG
      settings: MinAlgLoopOccurrences=on  RTWFcnNameOpts=User specified  RTWFileNameOpts=User specified
  Control_Commands : Outport
  Surf_saturated : Outport  Port=2
  Control_def for eval : Outport  Port=3

== system F16ASYM_Controlled/Environment params Estimations ==
  note: Acceleration of the body in body axes
  note: Acceleration of the body
      |   in wind axes
  All_meas : Inport
  ALT_and_M_GAIN_LIST : Gain
  A_b_CG : Product  Multiplication=Matrix(*)
  A_w_CG : Product  Multiplication=Matrix(*)
  Bias : Bias  Bias=-[0;0;1]
  Bus Creator : BusCreator  Inputs=8
  Bus Selector : BusSelector  OutputSignals=V_TAS (m/s),Alt meas (m),AoA meas (rad),SS meas (rad),Euler meas (rad),an_b_CG meas (m/s^2)
  Constant : Constant  Value=0
  Direction Cosine Matrix Body to Wind T_F_b->F_w : aerolibtransform2/Direction Cosine Matrix Body to Wind
  Divide : Product  Inputs=**
  Gain : Gain  Gain=1/2
  Gain1 : Gain  Gain=-1*9.81
  Gain2 : Gain  Gain=-1
  Gain3 : Gain  Gain=-1
  ISA Atmosphere Model : aerolibatmos2/ISA Atmosphere Model  custom=off  g=9.80665  gamma=1.4  R=287.0531  L=0.0065  h_trop=11000  h_strat=20000  rho0=1.225  P0=101325  T0=288.15  h0=0
  Mach number : Subsystem
  Matrix Multiply1 : Product  Multiplication=Matrix(*)
  Mux : Mux  Inputs=2
  Mux1 : Mux  Inputs=3
  Mux2 : Mux  Inputs=2
  Rotation Angles to Direction Cosine Matrix: F_b->F_T : aerolibtransform2/Rotation Angles to Direction Cosine Matrix  rotationOrder=ZYX
  Rotation Angles to Direction Cosine Matrix: F_h->F_b : aerolibtransform2/Rotation Angles to Direction Cosine Matrix  rotationOrder=ZYX
  Selector1 : Selector  InputPortWidth=3  Indices=[3 2 1]
  Selector7 : Selector  InputPortWidth=3  Indices=[3 2 1]
  Terminator : Terminator
  Terminator1 : Terminator
  Terminator2 : Terminator
  Transpose : Math  Operator=transpose  SaturateOnIntegerOverflow=on
  dyn pressure : Product  Inputs=**
  Params : Outport
  wires:
  All_meas/1 -> Bus Selector/1
  Bus Selector/1 -> Mach number/1(V), Divide/1, Divide/2  "<V_TAS (m/s)>"
  Bus Selector/2 -> Mux2/1, ISA Atmosphere Model/1  "<Alt meas (m)>"
  ISA Atmosphere Model/4 -> dyn pressure/2
  dyn pressure/1 -> Bus Creator/1  "q (Pa)"
  Bus Creator/1 -> Params/1
  Divide/1 -> Gain/1
  Gain/1 -> dyn pressure/1
  Bus Selector/3 -> Mux/1, Gain2/1  "<AoA meas (rad)>"
  Bus Selector/4 -> Gain3/1, Mux/2  "<SS meas (rad)>"
  Mux/1 -> Direction Cosine Matrix Body to Wind T_F_b->F_w/1
  Bus Selector/6 -> Matrix Multiply1/2  "<an_b_CG meas (m/s^2)>"
  Bus Selector/5 -> Selector7/1  "<Euler meas (rad)>"
  Selector7/1 -> Rotation Angles to Direction Cosine Matrix: F_h->F_b/1
  Rotation Angles to Direction Cosine Matrix: F_h->F_b/1 -> Transpose/1, Bus Creator/8, A_b_CG/1  "T_F_h->F_b"
  Matrix Multiply1/1 -> Bias/1
  Transpose/1 -> Matrix Multiply1/1
  Bias/1 -> Gain1/1
  A_b_CG/1 -> Bus Creator/7, A_w_CG/2  "A_b_CG"
  A_w_CG/1 -> Bus Creator/6  "A_w_CG"
  Gain1/1 -> A_b_CG/2
  Direction Cosine Matrix Body to Wind T_F_b->F_w/1 -> A_w_CG/1, Bus Creator/5  "T_F_b->F_w"
  Selector1/1 -> Rotation Angles to Direction Cosine Matrix: F_b->F_T/1
  Rotation Angles to Direction Cosine Matrix: F_b->F_T/1 -> Bus Creator/4  "T_F_b->F_T"
  Gain2/1 -> Mux1/1
  Gain3/1 -> Mux1/3
  Constant/1 -> Mux1/2
  Mux1/1 -> Selector1/1
  ISA Atmosphere Model/2 -> Bus Creator/3, Mach number/2(a)  "a"
  Mach number/1(Mach) -> Mux2/2, Bus Creator/2  "Mach"
  ISA Atmosphere Model/1 -> Terminator/1
  ISA Atmosphere Model/3 -> Terminator1/1  "Pressure (Pa)"
  Mux2/1 -> ALT_and_M_GAIN_LIST/1
  ALT_and_M_GAIN_LIST/1 -> Terminator2/1

== system F16ASYM_Controlled/F-16 Non-linear Plant ==
  States : Inport
  Reconf params : Inport  Port=2
  Control Comands : Inport  Port=3
  SYM and ASYM model: No reconfigurable : Subsystem  VariantControl=No Reconfigurable
  SYM and ASYM model: RECONFIGURABLE : Subsystem  VariantControl=Reconfigurable
  Output_bus : Outport
  Actual control def : Outport  Port=2

== system F16ASYM_Controlled/Faults injection ==
  note: Blockades now:
      | Input 1 to fixed controller at the current position
      | 0 otherwise
  note: Blockades: Input any number to fixed the
      | surface there. If non NaN
  note: RECONFIGURATION PARAMETERS
      |
      | 24. mass  Estimated mass
      | 25. S_current_L
      | 26. S_current_R
      | 27. S_fin_current
      | 28. x_cg
      | 29. Jy
      | 30. Jxz
      | 31. Jz
      | 32. Jx
      | 33. EFF_el_L
      | 34. EFF_el_R
      | 35. EFF_ail_L
      | 36. EFF_ail_R
      | 37. EFF_rud
      | 38. EFF_lef_L
      | 39. EFF_lef_R
      | 40. Delta_C_Lift_X
      | 41. Delta_C_Drag_X
      | 42. Delta_C_m_X
  Add : Sum
  Blockades at : Constant  Value="[NaN  NaN  NaN  NaN  NaN  NaN  NaN]"  SampleTime=T_sim
  Blockades now : Constant  Value="[0  0  0  0  0  0  0]"  SampleTime=T_sim
  Bus Creator : BusCreator  Inputs=3
  Delta_J : Constant  Value="[0  0  0  0]"  SampleTime=T_sim
  Gain : Gain  Gain="-[0  0  0  1  0  0  0]"
  MATLAB Function : MATLAB Function  TreatAsAtomicUnit=on
  Step : Step  Time=3  SampleTime=0
  Transpose : Math  Operator=transpose  SaturateOnIntegerOverflow=on
  delta_S_L : Constant  Value=[0]  SampleTime=T_sim
  delta_S_R : Constant  Value=[0]  SampleTime=T_sim
  delta_S_fin : Constant  Value=[0]  SampleTime=T_sim
  delta_coef : Constant  Value="[0  0  0]"  SampleTime=T_sim
  delta_mass : Constant  Value=[0]  SampleTime=T_sim
  effectiveness : Constant  Value="[1  1  1  1  1  1  1]"  SampleTime=T_sim
  xcg : Constant  Value=[0.3]  SampleTime=T_sim
  Reconf bus : Outport
  wires:
  MATLAB Function/1(reconfig_params) -> Bus Creator/1  "Reconfig signal"
  Bus Creator/1 -> Reconf bus/1
  Blockades at/1 -> Bus Creator/2  "Blockades"
  Transpose/1 -> Bus Creator/3  "Blockade now"
  delta_mass/1 -> MATLAB Function/1(Delta_mass)
  delta_S_L/1 -> MATLAB Function/2(Delta_S_L)
  delta_S_R/1 -> MATLAB Function/3(Delta_S_R)
  delta_S_fin/1 -> MATLAB Function/4(Delta_S_Fin)
  xcg/1 -> MATLAB Function/5(xcg)
  Delta_J/1 -> MATLAB Function/6(Delta_J)
  Add/1 -> MATLAB Function/7(Eff)
  delta_coef/1 -> MATLAB Function/8(Deltas_coef)
  Step/1 -> Gain/1
  Blockades now/1 -> Transpose/1
  Gain/1 -> Add/2
  effectiveness/1 -> Add/1

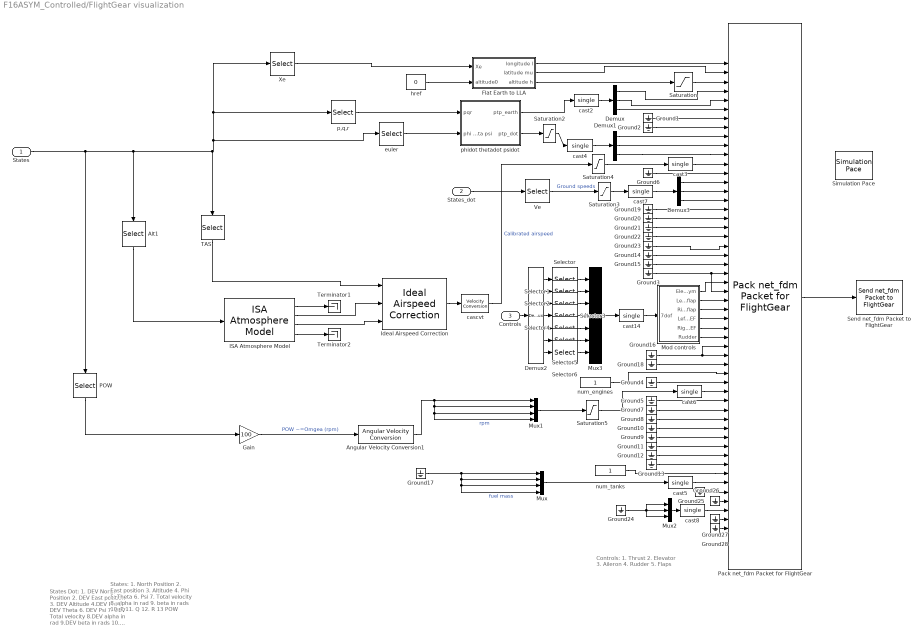
== system F16ASYM_Controlled/FlightGear visualization ==
  note: States Dot:
      | 1. DEV North Position
      | 2. DEV East position
      | 3. DEV Altitude
      | 4.DEV  Phi
      | 5. DEV Theta
      | 6. DEV Psi
      | 7. DEV Total velocity
      | 8.DEV alpha in rad
      | 9.DEV  beta in rads
      | 10. DEV P
      | 11. DEV Q
      | 12. DEV R
  note: States:
      | 1. North Position
      | 2. East position
      | 3. Altitude
      | 4. Phi
      | 5. Theta
      | 6. Psi
      | 7. Total velocity
      | 8. alpha in rad
      | 9. beta in rads
      | 10. P
      | 11. Q
      | 12. R
      | 13 POW
  note: Controls:
      | 1. Thrust
      | 2. Elevator
      | 3. Aileron
      | 4. Rudder
      | 5. Flaps
  States : Inport
  States_dot : Inport  Port=2
  Controls : Inport  Port=3
  Alt1 : Selector  InputPortWidth=13  Indices=3
  Angular Velocity Conversion1 : aerolibconvert2/Angular Velocity Conversion  IU=rad/s  OU=rpm
  Demux : Demux  Outputs=3
  Demux1 : Demux  Outputs=3
  Demux2 : Demux  Outputs=7
  Demux3 : Demux  Outputs=3
  Flat Earth to LLA : Subsystem
  Gain : Gain  Gain=100
  Ground{1..28} (28 alike) : Ground
  ISA Atmosphere Model : aerolibatmos2/ISA Atmosphere Model  custom=off  g=9.80665  gamma=1.4  R=287.0531  L=0.0065  h_trop=11000  h_strat=20000  rho0=1.225  P0=101325  T0=288.15  h0=0
  Ideal Airspeed Correction : aerolibasang/Ideal Airspeed Correction  units=Metric (MKS)  vel_in=TAS  vel_out_tas=CAS  vel_out_eas=CAS  vel_out_cas=TAS  action=None
  Mod controls : Subsystem  TreatAsAtomicUnit=on
  Mux : Mux
  Mux1 : Mux
  Mux2 : Mux  Inputs=3
  Mux3 : Mux  Inputs=7
  POW : Selector  InputPortWidth=13  Indices=13
  Pack net_fdm Packet for FlightGear : aerolibfltsims/Pack net_fdm Packet for FlightGear  FlightGearVersion=v2.0  ShowPositionAttitudeInputs=on  ShowVelocityAccelerationInputs=on  ShowControlSurfacePositionInputs=on  ShowEngineFuelInputs=on  ShowLandingGearInputs=on  ShowEnvironmentInputs=off  SampleTime=-1
      settings: AttributesFormatString=FG VERSION: %<FlightGearVersion>
  Saturation : Saturate  UpperLimit=1e8  LowerLimit=-1e5
  Saturation2 : Saturate  UpperLimit=1e3  LowerLimit=-1e3
  Saturation3 : Saturate  UpperLimit=1e4  LowerLimit=-1e4
  Saturation4 : Saturate  UpperLimit=1e4  LowerLimit=-1e4
  Saturation5 : Saturate  UpperLimit=1e6  LowerLimit=0
  Selector{,1..6} (7 alike) : Selector  InputPortWidth=2  Indices=2
  Send net_fdm Packet to FlightGear : aerolibfltsims/Send net_fdm Packet to FlightGear  DestinationIpAddress=127.0.0.1  DestinationPort=5502  LocalIpPort=-1  varLen=off  SampleTime=-1
  Simulation Pace : aerolibanimutils/Simulation Pace  SimulationPace=1  SleepMode=MATLAB Thread  OutputPaceError=off  SampleTime=4*T_sim
      settings: AttributesFormatString=%<SimulationPace> sec/sec
  TAS : Selector  InputPortWidth=13  Indices=7
  Terminator1 : Terminator
  Terminator2 : Terminator
  Ve : Selector  InputPortWidth=13  Indices=[1:3]
  Xe : Selector  InputPortWidth=13  Indices=[1:3]
  cascvt : aerolibconvert/Velocity Conversion  IU=m/s  OU=kts
  cast{2..8,14} (8 alike) : DataTypeConversion  OutDataTypeStr=single  SaturateOnIntegerOverflow=on
  euler : Selector  InputPortWidth=13  Indices=[4:6]
  href : Constant  Value=0  VectorParams1D=off
  num_engines : Constant  OutDataTypeStr=uint32
  num_tanks : Constant  OutDataTypeStr=uint32
  p,q,r : Selector  InputPortWidth=13  Indices=[10:12]
  phidot thetadot psidot : Subsystem
  wires:
  Pack net_fdm Packet for FlightGear/1 -> Send net_fdm Packet to FlightGear/1
  Ground3/1 -> Pack net_fdm Packet for FlightGear/24, Pack net_fdm Packet for FlightGear/26
  Demux1/3 -> Pack net_fdm Packet for FlightGear/11
  Demux1/2 -> Pack net_fdm Packet for FlightGear/10
  Demux1/1 -> Pack net_fdm Packet for FlightGear/9
  Ground2/1 -> Pack net_fdm Packet for FlightGear/8
  Ground1/1 -> Pack net_fdm Packet for FlightGear/7
  Demux/3 -> Pack net_fdm Packet for FlightGear/6
  Demux/2 -> Pack net_fdm Packet for FlightGear/5
  Demux/1 -> Pack net_fdm Packet for FlightGear/4
  Ground6/1 -> Pack net_fdm Packet for FlightGear/13
  ISA Atmosphere Model/2 -> Ideal Airspeed Correction/2
  phidot thetadot psidot/2(ptp_dot) -> Saturation2/1
  phidot thetadot psidot/1(ptp_earth) -> cast2/1
  cast3/1 -> Pack net_fdm Packet for FlightGear/12
  cascvt/1 -> Saturation4/1  "Calibrated airspeed"
  Ideal Airspeed Correction/1 -> cascvt/1
  Ground15/1 -> Pack net_fdm Packet for FlightGear/23
  Ground14/1 -> Pack net_fdm Packet for FlightGear/22
  Ground23/1 -> Pack net_fdm Packet for FlightGear/21
  Ground22/1 -> Pack net_fdm Packet for FlightGear/20
  Ground21/1 -> Pack net_fdm Packet for FlightGear/19
  Ground20/1 -> Pack net_fdm Packet for FlightGear/18
  Ground19/1 -> Pack net_fdm Packet for FlightGear/17
  href/1 -> Flat Earth to LLA/2(altitude0)
  Flat Earth to LLA/3(altitude h) -> Saturation/1
  States/1 -> p,q,r/1, Xe/1, euler/1, TAS/1, Alt1/1, POW/1
  Flat Earth to LLA/1(longitude l) -> Pack net_fdm Packet for FlightGear/1
  Flat Earth to LLA/2(latitude mu) -> Pack net_fdm Packet for FlightGear/2
  Demux3/1 -> Pack net_fdm Packet for FlightGear/14
  Demux3/2 -> Pack net_fdm Packet for FlightGear/15
  Demux3/3 -> Pack net_fdm Packet for FlightGear/16
  Ve/1 -> Saturation3/1  "Ground speeds"
  cast2/1 -> Demux/1
  cast4/1 -> Demux1/1
  cast5/1 -> Pack net_fdm Packet for FlightGear/47
  cast6/1 -> Pack net_fdm Packet for FlightGear/37
  num_tanks/1 -> Pack net_fdm Packet for FlightGear/46
  ISA Atmosphere Model/1 -> Terminator1/1
  ISA Atmosphere Model/4 -> Terminator2/1
  ISA Atmosphere Model/3 -> Ideal Airspeed Correction/3
  Alt1/1 -> ISA Atmosphere Model/1
  Ground17/1 -> Mux/2, Mux/3, Mux/4, Mux/1  "fuel mass"
  Mux/1 -> cast5/1
  Gain/1 -> Angular Velocity Conversion1/1  "POW ~=Omgea (rpm)"
  Mux1/1 -> Saturation5/1
  cast7/1 -> Demux3/1
  Angular Velocity Conversion1/1 -> Mux1/2, Mux1/3, Mux1/4, Mux1/1  "rpm"
  Saturation/1 -> Pack net_fdm Packet for FlightGear/3
  Saturation2/1 -> cast4/1
  Saturation3/1 -> cast7/1
  Saturation4/1 -> cast3/1
  Saturation5/1 -> cast6/1
  States_dot/1 -> Ve/1
  Ground5/1 -> Pack net_fdm Packet for FlightGear/38
  Ground7/1 -> Pack net_fdm Packet for FlightGear/39
  Ground8/1 -> Pack net_fdm Packet for FlightGear/40
  Ground10/1 -> Pack net_fdm Packet for FlightGear/41
  Ground9/1 -> Pack net_fdm Packet for FlightGear/42
  Ground11/1 -> Pack net_fdm Packet for FlightGear/43
  Ground12/1 -> Pack net_fdm Packet for FlightGear/44
  Ground13/1 -> Pack net_fdm Packet for FlightGear/45
  Ground4/1 -> Pack net_fdm Packet for FlightGear/36
  num_engines/1 -> Pack net_fdm Packet for FlightGear/35
  Controls/1 -> Demux2/1
  Ground18/1 -> Pack net_fdm Packet for FlightGear/34
  Ground16/1 -> Pack net_fdm Packet for FlightGear/32, Pack net_fdm Packet for FlightGear/33
  Xe/1 -> Flat Earth to LLA/1(Xe)
  euler/1 -> phidot thetadot psidot/2(phi theta psi)
  TAS/1 -> Ideal Airspeed Correction/1
  p,q,r/1 -> phidot thetadot psidot/1(pqr)
  POW/1 -> Gain/1
  Mux3/1 -> cast14/1
  Mod controls/1(Elevator Sym) -> Pack net_fdm Packet for FlightGear/25
  Ground24/1 -> Mux2/3, Mux2/2, Mux2/1
  cast8/1 -> Pack net_fdm Packet for FlightGear/50
  Mux2/1 -> cast8/1
  Demux2/1 -> Selector/1
  Demux2/2 -> Selector1/1
  Demux2/3 -> Selector2/1
  Demux2/4 -> Selector3/1
  Demux2/5 -> Selector4/1
  Demux2/6 -> Selector5/1
  Demux2/7 -> Selector6/1
  Selector/1 -> Mux3/1
  Selector1/1 -> Mux3/2
  Selector2/1 -> Mux3/3
  Selector3/1 -> Mux3/4
  Selector4/1 -> Mux3/5
  Selector5/1 -> Mux3/6
  Selector6/1 -> Mux3/7
  Ground25/1 -> Pack net_fdm Packet for FlightGear/48
  Ground26/1 -> Pack net_fdm Packet for FlightGear/49
  Ground27/1 -> Pack net_fdm Packet for FlightGear/51
  Ground28/1 -> Pack net_fdm Packet for FlightGear/52
  Mod controls/3(Right flap) -> Pack net_fdm Packet for FlightGear/28
  Mod controls/4(Left LEF) -> Pack net_fdm Packet for FlightGear/29
  Mod controls/5(Right LEF) -> Pack net_fdm Packet for FlightGear/30
  Mod controls/6(Rudder) -> Pack net_fdm Packet for FlightGear/31
  Mod controls/2(Left flap) -> Pack net_fdm Packet for FlightGear/27
  cast14/1 -> Mod controls/1("7dof ")

== system F16ASYM_Controlled/Inject Failures and NN ==

== system F16ASYM_Controlled/NDI ==
  Est reconf : Inport
  Angular_acc_des (rad/s^2) : Inport  Port=2
  All_meas : Inport  Port=3
  Control_defl for eval : Inport  Port=4
  NDI: NO RECONFIG : Subsystem  RTWFcnName=abc  RTWFileName=asas  VariantControl=NDI: NO RECONFIG
      settings: RTWFcnNameOpts=User specified  RTWFileNameOpts=User specified
  NDI: RECONFIG : Subsystem  RTWFcnName=abc  RTWFileName=asas  VariantControl=NDI: RECONFIG
      settings: RTWFcnNameOpts=User specified  RTWFileNameOpts=User specified
  Virtual Control Commands : Outport
  B online : Outport  Port=2
  Control_defl evald : Outport  Port=3
  Mom coef comm : Outport  Port=4
